simulink model "ControlMRAC"  (R2022b)
settings: Solver=ode4  StartTime=0.0  StopTime=60  FixedStep=.001  RelTol=1e-3
values from neighbouring files (symbols this model uses):
  B = [zeros(n,n);eye(n,n)]    [IniciadorParametros.m]
  Psi1 = [V1 zeros(n,n)]    [IniciadorParametros.m]
  Psi2 = [zeros(n,n) V2]    [IniciadorParametros.m]
  V0 = Data(:,1)    [IniciadorParametros.m]
undefined symbols (not defined in the file or in its folder): A, Gamma, P, W1, W2
settings Model: Creator=raul  LastModifiedBy=raul

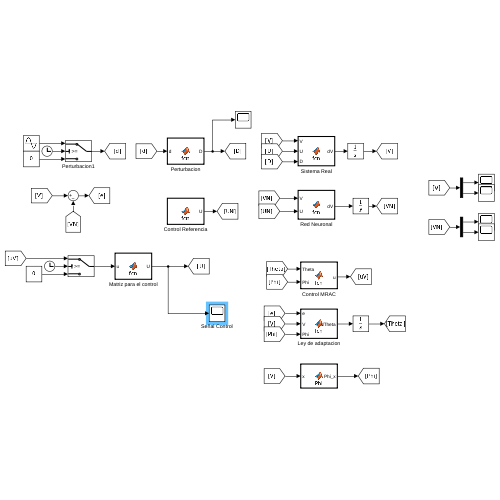
[thumbnail: Simulink's stored preview of the top-level diagram]
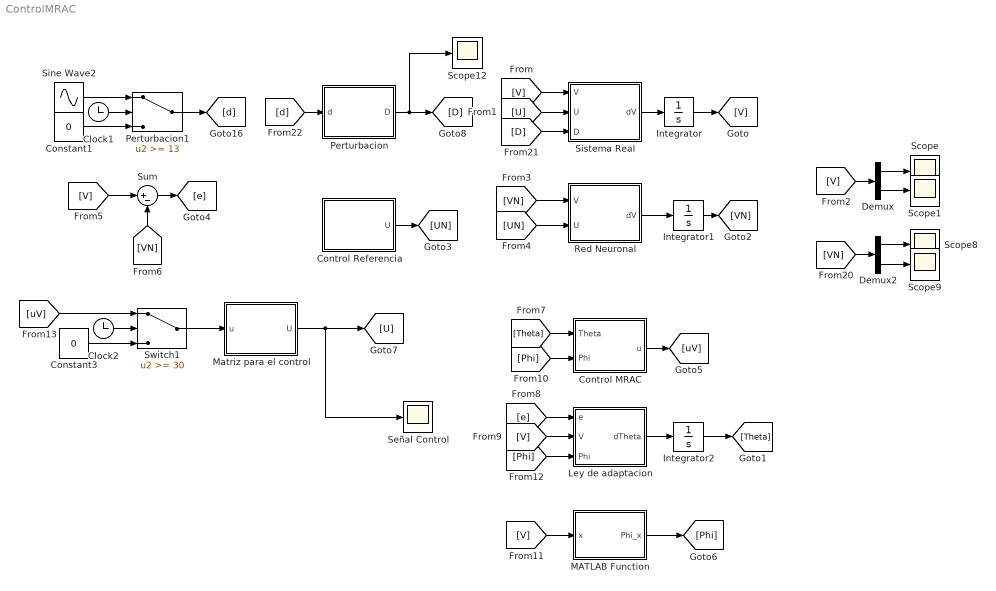
== system ControlMRAC ==
  Clock1 : Clock
  Clock2 : Clock
  Constant1 : Constant  Value=0
  Constant3 : Constant  Value=0
  Control MRAC : MATLAB Function  TreatAsAtomicUnit=on
  Control Referencia : MATLAB Function  TreatAsAtomicUnit=on
  Demux : Demux  Outputs=2
  Demux2 : Demux  Outputs=2
  Integrator : Integrator  InitialCondition=V0
  Integrator1 : Integrator  InitialCondition=V0
  Integrator2 : Integrator  InitialCondition=zeros(20,1)
  Ley de adaptacion : MATLAB Function  TreatAsAtomicUnit=on
  MATLAB Function : MATLAB Function  TreatAsAtomicUnit=on
  Matriz para el control : MATLAB Function  TreatAsAtomicUnit=on
  Perturbacion : MATLAB Function  TreatAsAtomicUnit=on
  Perturbacion1 : Switch  Threshold=13  SaturateOnIntegerOverflow=off  InputSameDT=off
  Red Neuronal : MATLAB Function  TreatAsAtomicUnit=on
  Scope{,1,8..9,12} (5 alike) : Scope
  Señal Control : Scope
  Sine Wave2 : Sin  Frequency=5  SampleTime=0
  Sistema Real : MATLAB Function  TreatAsAtomicUnit=on
  Sum : Sum  Inputs=|+-
  Switch1 : Switch  Threshold=30  SaturateOnIntegerOverflow=off  InputSameDT=off
  wires:
  [V] -> Demux/1
  Demux/1 -> Scope/1
  [d] -> Perturbacion/1(d)
  [V] -> Sistema Real/1(V)
  Integrator/1 -> [V]
  Sistema Real/1(dV) -> Integrator/1
  [U] -> Sistema Real/2(U)
  [VN] -> Demux2/1
  Demux2/2 -> Scope9/1
  Perturbacion/1(D) -> Scope12/1, [D]
  [D] -> Sistema Real/3(D)
  Demux/2 -> Scope1/1
  Demux2/1 -> Scope8/1
  Perturbacion1/1 -> [d]
  Sine Wave2/1 -> Perturbacion1/1
  Clock1/1 -> Perturbacion1/2
  Constant1/1 -> Perturbacion1/3
  Sum/1 -> [e]
  [V] -> Sum/1
  [VN] -> Sum/2
  Control Referencia/1(U) -> [UN]
  [UN] -> Red Neuronal/2(U)
  Integrator1/1 -> [VN]
  Red Neuronal/1(dV) -> Integrator1/1
  [VN] -> Red Neuronal/1(V)
  Ley de adaptacion/1(dTheta) -> Integrator2/1
  Integrator2/1 -> [Theta]
  [Theta] -> Control MRAC/1(Theta)
  Control MRAC/1(u) -> [uV]
  [e] -> Ley de adaptacion/1(e)
  [V] -> Ley de adaptacion/2(V)
  Clock2/1 -> Switch1/2
  Switch1/1 -> Matriz para el control/1(u)
  Constant3/1 -> Switch1/3
  [uV] -> Switch1/1
  Matriz para el control/1(U) -> Señal Control/1, [U]
  [Phi] -> Control MRAC/2(Phi)
  [V] -> MATLAB Function/1(x)
  MATLAB Function/1(Phi_x) -> [Phi]
  [Phi] -> Ley de adaptacion/3(Phi)

== matlab function ControlMRAC/Control MRAC ==
  data: Theta input; u output; Phi input
function u = fcn(Theta, Phi)


% alpha = 1 - exp(-0.1 * (t - 30)); % Transición suave después de t=30
u = - Theta' * Phi;


end

== matlab function ControlMRAC/Sistema Real ==
  data: V input; U input; dV output; W1 parameter; W2 parameter; Psi1 parameter; Psi2 parameter; B parameter; A parameter; D input
function dV  = fcn(V, U, W1, W2, Psi1, Psi2, B, A,D)

dV=A*V+B*(W1*sigmoid(Psi1,V)+W2*phi_sigmoid(Psi2,V)*U+W2*phi_sigmoid(Psi2,V)*D);


function s = sigmoid(b,x)
   s = 1./(1+exp(-b*x)); 
end



function phi = phi_sigmoid(bp, xp)
    % Comprueba que b y x tengan las dimensiones adecuadas
    [rows_b, cols_b] = size(bp);
%     [rows_x, cols_x] = size(xp);

    % Inicializa la matriz de salida
    phi = zeros(rows_b, rows_b); % Matriz de 20x20

    % Calcula la sigmoide combinando cada fila de b con el vector x
    for i = 1:rows_b
        phi(i, :) = 1 ./ (1 + exp(-bp(i, :) * xp)); % Producto y sigmoide
    end
end



end

== matlab function ControlMRAC/Red Neuronal ==
  data: V input; U input; dV output; W1 parameter; W2 parameter; Psi1 parameter; Psi2 parameter; B parameter; A parameter
function dV  = fcn(V, U, W1, W2, Psi1, Psi2, B, A)

dV=A*V+B*(W1*sigmoid(Psi1,V)+W2*phi_sigmoid(Psi2,V)*U);


function s = sigmoid(b,x)
   s = 1./(1+exp(-b*x)); 
end



function phi = phi_sigmoid(bp, xp)
    % Comprueba que b y x tengan las dimensiones adecuadas
    [rows_b, cols_b] = size(bp);
%     [rows_x, cols_x] = size(xp);

    % Inicializa la matriz de salida
    phi = zeros(rows_b, rows_b); % Matriz de 20x20

    % Calcula la sigmoide combinando cada fila de b con el vector x
    for i = 1:rows_b
        phi(i, :) = 1 ./ (1 + exp(-bp(i, :) * xp)); % Producto y sigmoide
    end
end



end

== matlab function ControlMRAC/Ley de adaptacion ==
  data: e input; dTheta output; Gamma parameter; P parameter; V input; Psi2 parameter; W2 parameter; Phi input
function dTheta = fcn(e, Gamma, P, V, Psi2, W2,Phi)
e_s=e(1:20);
B=W2*sigmoid(Psi2,V);

dTheta = -Gamma*Phi*e_s'*P*B;


function s = sigmoid(b,x)
   s = 1./(1+exp(-b*x)); 
end





end

== matlab function ControlMRAC/Control Referencia ==
  data: U output
function U = fcn()%add Bw,w

U=zeros(20,1);

== matlab function ControlMRAC/Matriz para el control ==
  data: U output; u input; nodeControl parameter
function U = fcn(u, nodeControl)%add Bw,w

U=zeros(20,1);
U(nodeControl,1)=u;

== matlab function ControlMRAC/Perturbacion ==
  data: D output; d input; nodeDisturbe parameter
function D = fcn(d, nodeDisturbe)%add Bw,w

D=zeros(20,1);
D(nodeDisturbe,1)=d;

== matlab function ControlMRAC/MATLAB Function ==
  data: x input; Phi_x output
function Phi_x = Phi(x)
    % x es un vector de tamaño (20x1), representa los estados que controlamos
    Phi_x = zeros(20,1);
    
    % Para cada nodo, usar senos y cosenos de su posición
    for i = 1:10 % Solo iteramos sobre los primeros 10 nodos
        Phi_x(2*i-1) = sin(x(i))*cos(x(i));  % Componente impar -> sin(x)
        Phi_x(2*i) = sin(x(i))*cos(x(i));    % Componente par -> cos(x)
    end
end
